simulink model "DCMOTOR"  (R2025a)
settings: Solver=VariableStepAuto  StartTime=0.0  StopTime=10.0  RelTol=1e-3
libraries: simulink_extras x2
settings Model: Creator=gades  LastModifiedBy=gades

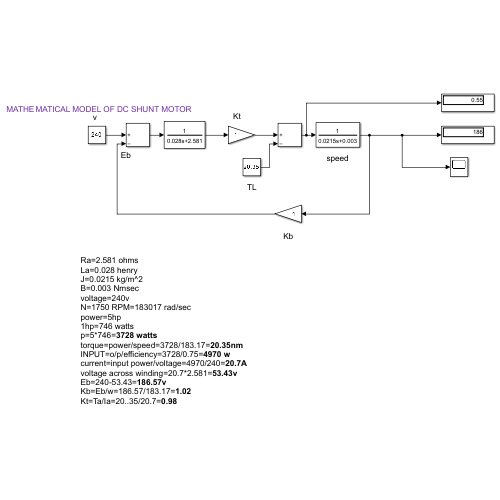
[thumbnail: Simulink's stored preview of the top-level diagram]
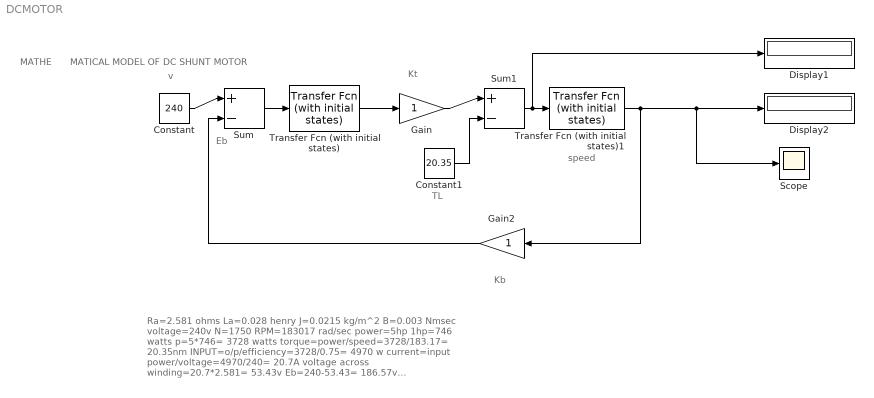
== system DCMOTOR ==
  note: MATICAL MODEL OF DC SHUNT MOTOR
  note: MATHE
  note: Ra=2.581 ohms
      | La=0.028 henry
      | J=0.0215 kg/m^2
      | B=0.003 Nmsec
      | voltage=240v
      | N=1750 RPM=183017 rad/sec
      | power=5hp
      | 1hp=746 watts
      | p=5*746= 3728 watts
      | torque=power/speed=3728/183.17= 20.35nm
      | INPUT=o/p/efficiency=3728/0.75= 4970 w
      | current=input power/voltage=4970/240= 20.7A
      | voltage across winding=20.7*2.581= 53.43v
      | Eb=240-53.43= 186.57v
      | Kb=Eb/w=186.57/183.17= 1.02
      | Kt=Ta/Ia=20..35/20.7= 0.98
  note: speed
  note: v
  note: Eb
  note: TL
  note: Kb
  note: Kt
  Constant : Constant  Value=240
  Constant1 : Constant  Value=20.35
  Display1 : Display
  Display2 : Display
  Gain : Gain
  Gain2 : Gain
  Scope : Scope
  Sum : Sum  Inputs=|+-
  Sum1 : Sum  Inputs=|+-
  Transfer Fcn (with initial states) : simulink_extras/Additional Linear/Transfer Fcn (with initial states)  N=[1]  D=[0.028 2.581]  X0=.5
  Transfer Fcn (with initial states)1 : simulink_extras/Additional Linear/Transfer Fcn (with initial states)  N=[1]  D=[0.0215 0.003]  X0=.5
  wires:
  Constant/1 -> Sum/1
  Sum/1 -> Transfer Fcn (with initial states)/1
  Transfer Fcn (with initial states)/1 -> Gain/1
  Gain/1 -> Sum1/1
  Transfer Fcn (with initial states)1/1 -> Gain2/1, Scope/1, Display2/1
  Gain2/1 -> Sum/2
  Constant1/1 -> Sum1/2
  Sum1/1 -> Transfer Fcn (with initial states)1/1, Display1/1
